simulink library "TM_MASTER"  (Simulink 8.6)
settings: Solver=ode45  StartTime=0.0  StopTime=10.0  RelTol=1e-3
libraries: cdsFilt x75, VIS_LIB x63, cdsEpicsOut x60, cdsTP x48, cdsMuxMatrix x17, cdsFiltCtrl x15, lockin x10, QPD x10, cdsRms x6, FOUROSEM_COILOUTF_MASTER x5, cdsFunctionCall x5, CRYP_TM_MASTER x3
(part 8 of 9)

== system TM_MASTER/TM_TYPEBP/ADD ==
  ISC_L_In : Inport
  ISC_P_In : Inport  Port=2
  ISC_Y_In : Inport  Port=3
  TEST_L_In : Inport  Port=4
  TEST_P_In : Inport  Port=5
  TEST_Y_In : Inport  Port=6
  DAMP_L_In : Inport  Port=7
  DAMP_P_In : Inport  Port=8
  DAMP_Y_In : Inport  Port=9
  Ground{1..6} (6 alike) : Ground
  L : cdsFiltCtrl/IIR FM with control  Tag=cdsFiltCtrl  Description=|
      | cdsFiltCntrl is the standard IIR filter module (exactly the same as cdsFilt) but with added control data output 'Ctrl'. Filter module digital signal output appears on the first output, which is called 'Val'. 'Ctrl' output has a bit pattern encoding the state of filter's on/off switches (FM1 through FM10). The bit values are:
      |                                                                                                                                                                                                                                                                                                                                       
      | module 	hex	dec                                                                                                                                                                                                                                                                                                                       
      | -----------------------                                                                                                                                                                                                                                                                                                               
      | FM1	0x20                    32                                                                                                                                                                                                                                                                                                        
      | FM2	0x80                     128                                                                                                                                                                                                                                                                                                      
      | FM3	0x200                   512                                                                                                                                                                                                                                                                                                       
      | FM4	0x800                   2048                                                                                                                                                                                                                                                                                                      
      | FM5	0x2000                 8192                                                                                                                                                                                                                                                                                                       
      | FM6	0x8000                 32768                                                                                                                                                                                                                                                                                                      
      | FM7	0x20000                131072                                                                                                                                                                                                                                                                                                     
      | FM8	0x80000                 524288                                                                                                                                                                                                                                                                                                    
      | FM9	0x200000               2097152                                                                                                                                                                                                                                                                                                    
      | FM10	0x800000               8388608                                                                                                                                                                                                                                                                                                   
      |                                                                                                                                                                                                                                                                                                                                       
      | This bit data can be used to drive some other switches or it can be output using a binary I/O module.
      settings: AttributesFormatString=%<Tag>
  P : cdsFiltCtrl/IIR FM with control  Tag=cdsFiltCtrl  Description=|
      | cdsFiltCntrl is the standard IIR filter module (exactly the same as cdsFilt) but with added control data output 'Ctrl'. Filter module digital signal output appears on the first output, which is called 'Val'. 'Ctrl' output has a bit pattern encoding the state of filter's on/off switches (FM1 through FM10). The bit values are:
      |                                                                                                                                                                                                                                                                                                                                       
      | module 	hex	dec                                                                                                                                                                                                                                                                                                                       
      | -----------------------                                                                                                                                                                                                                                                                                                               
      | FM1	0x20                    32                                                                                                                                                                                                                                                                                                        
      | FM2	0x80                     128                                                                                                                                                                                                                                                                                                      
      | FM3	0x200                   512                                                                                                                                                                                                                                                                                                       
      | FM4	0x800                   2048                                                                                                                                                                                                                                                                                                      
      | FM5	0x2000                 8192                                                                                                                                                                                                                                                                                                       
      | FM6	0x8000                 32768                                                                                                                                                                                                                                                                                                      
      | FM7	0x20000                131072                                                                                                                                                                                                                                                                                                     
      | FM8	0x80000                 524288                                                                                                                                                                                                                                                                                                    
      | FM9	0x200000               2097152                                                                                                                                                                                                                                                                                                    
      | FM10	0x800000               8388608                                                                                                                                                                                                                                                                                                   
      |                                                                                                                                                                                                                                                                                                                                       
      | This bit data can be used to drive some other switches or it can be output using a binary I/O module.
      settings: AttributesFormatString=%<Tag>
  Sum : Sum  Inputs=+++
  Sum3 : Sum  Inputs=+++
  Sum4 : Sum  Inputs=+++
  Terminator1 : Terminator
  Terminator2 : Terminator
  Terminator3 : Terminator
  Y : cdsFiltCtrl/IIR FM with control  Tag=cdsFiltCtrl  Description=|
      | cdsFiltCntrl is the standard IIR filter module (exactly the same as cdsFilt) but with added control data output 'Ctrl'. Filter module digital signal output appears on the first output, which is called 'Val'. 'Ctrl' output has a bit pattern encoding the state of filter's on/off switches (FM1 through FM10). The bit values are:
      |                                                                                                                                                                                                                                                                                                                                       
      | module 	hex	dec                                                                                                                                                                                                                                                                                                                       
      | -----------------------                                                                                                                                                                                                                                                                                                               
      | FM1	0x20                    32                                                                                                                                                                                                                                                                                                        
      | FM2	0x80                     128                                                                                                                                                                                                                                                                                                      
      | FM3	0x200                   512                                                                                                                                                                                                                                                                                                       
      | FM4	0x800                   2048                                                                                                                                                                                                                                                                                                      
      | FM5	0x2000                 8192                                                                                                                                                                                                                                                                                                       
      | FM6	0x8000                 32768                                                                                                                                                                                                                                                                                                      
      | FM7	0x20000                131072                                                                                                                                                                                                                                                                                                     
      | FM8	0x80000                 524288                                                                                                                                                                                                                                                                                                    
      | FM9	0x200000               2097152                                                                                                                                                                                                                                                                                                    
      | FM10	0x800000               8388608                                                                                                                                                                                                                                                                                                   
      |                                                                                                                                                                                                                                                                                                                                       
      | This bit data can be used to drive some other switches or it can be output using a binary I/O module.
      settings: AttributesFormatString=%<Tag>
  LONG_Out : Outport
  PITCH_Out : Outport  Port=2
  YAW_Out : Outport  Port=3
  wires:
  Y/2 -> Terminator3/1
  P/2 -> Terminator2/1
  L/2 -> Terminator1/1
  Y/1 -> YAW_Out/1
  Ground5/1 -> Y/2
  Ground4/1 -> Y/3
  Sum3/1 -> Y/1
  P/1 -> PITCH_Out/1
  Ground3/1 -> P/2
  Ground2/1 -> P/3
  Sum4/1 -> P/1
  L/1 -> LONG_Out/1
  Ground6/1 -> L/2
  Ground1/1 -> L/3
  Sum/1 -> L/1
  ISC_P_In/1 -> Sum4/1
  TEST_P_In/1 -> Sum4/2
  TEST_Y_In/1 -> Sum3/2
  ISC_Y_In/1 -> Sum3/1
  TEST_L_In/1 -> Sum/2
  ISC_L_In/1 -> Sum/1
  DAMP_L_In/1 -> Sum/3
  DAMP_P_In/1 -> Sum4/3
  DAMP_Y_In/1 -> Sum3/3

== system TM_MASTER/TM_TYPEBP/ADDASC ==
  ISC_P_In : Inport
  ISC_Y_In : Inport  Port=2
  DITHER_P_In : Inport  Port=3
  DITHER_Y_In : Inport  Port=4
  Sum3 : Sum
  Sum4 : Sum
  PITCH_Out : Outport
  YAW_Out : Outport  Port=2
  wires:
  Sum3/1 -> YAW_Out/1
  ISC_P_In/1 -> Sum4/1
  ISC_Y_In/1 -> Sum3/1
  Sum4/1 -> PITCH_Out/1
  DITHER_P_In/1 -> Sum4/2
  DITHER_Y_In/1 -> Sum3/2

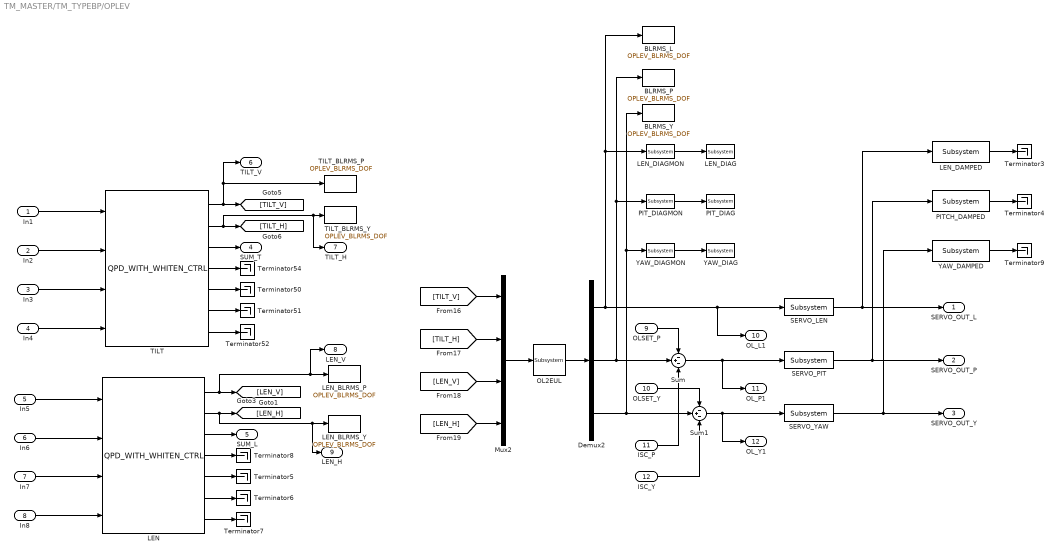
== system TM_MASTER/TM_TYPEBP/OPLEV ==
  In1 : Inport
  In2 : Inport  Port=2
  In3 : Inport  Port=3
  In4 : Inport  Port=4
  In5 : Inport  Port=5
  In6 : Inport  Port=6
  In7 : Inport  Port=7
  In8 : Inport  Port=8
  OLSET_P : Inport  Port=9
  OLSET_Y : Inport  Port=10
  ISC_P : Inport  Port=11
  ISC_Y : Inport  Port=12
  BLRMS_L : VIS_LIB/OPLEV_BLRMS_DOF
  BLRMS_P : VIS_LIB/OPLEV_BLRMS_DOF
  BLRMS_Y : VIS_LIB/OPLEV_BLRMS_DOF
  Demux2 : Demux  Outputs=3
  LEN : QPD/QPD_WITH_WHITEN_CTRL
  LEN_BLRMS_P : VIS_LIB/OPLEV_BLRMS_DOF
  LEN_BLRMS_Y : VIS_LIB/OPLEV_BLRMS_DOF
  LEN_DAMPED : cdsEpicsOut/Subsystem  Tag=cdsEpicsOutput  Description=|
      | Purpose:                                          
      | Output a FE signal to an EPICS channel.           
      |                                                   
      | Operation:                                        
      | Takes input value and passes it to EPICS record.  
      |                                                   
      | Usage:                                            
      | Name the part with the desired EPICS rrecord name.
      settings: AttributesFormatString=%<Tag>
  LEN_DIAG : cdsTP/Subsystem  Tag=Test Point
      settings: AttributesFormatString=%<Tag>
  LEN_DIAGMON : cdsEpicsOut/Subsystem  Tag=cdsEpicsOutput  Description=|
      | Purpose:                                          
      | Output a FE signal to an EPICS channel.           
      |                                                   
      | Operation:                                        
      | Takes input value and passes it to EPICS record.  
      |                                                   
      | Usage:                                            
      | Name the part with the desired EPICS rrecord name.
      settings: AttributesFormatString=%<Tag>
  Mux2 : Mux
  OL2EUL : cdsMuxMatrix/Subsystem  Tag=cdsMuxMatrix  Description=Any size matrix. Inputs and outputs must be connected using Mux and Demux parts.
      settings: AttributesFormatString=%<Tag>
  PITCH_DAMPED : cdsEpicsOut/Subsystem  Tag=cdsEpicsOutput  Description=|
      | Purpose:                                          
      | Output a FE signal to an EPICS channel.           
      |                                                   
      | Operation:                                        
      | Takes input value and passes it to EPICS record.  
      |                                                   
      | Usage:                                            
      | Name the part with the desired EPICS rrecord name.
      settings: AttributesFormatString=%<Tag>
  PIT_DIAG : cdsTP/Subsystem  Tag=Test Point
      settings: AttributesFormatString=%<Tag>
  PIT_DIAGMON : cdsEpicsOut/Subsystem  Tag=cdsEpicsOutput  Description=|
      | Purpose:                                          
      | Output a FE signal to an EPICS channel.           
      |                                                   
      | Operation:                                        
      | Takes input value and passes it to EPICS record.  
      |                                                   
      | Usage:                                            
      | Name the part with the desired EPICS rrecord name.
      settings: AttributesFormatString=%<Tag>
  SERVO_LEN : cdsFilt/Subsystem  Tag=cdsFilt  Description=|
      | Purpose:                                                                                                                                                                                                                                  
      | Standard CDS IIR filter module.                                                                                                                                                                                                           
      |                                                                                                                                                                                                                                           
      | Operation:                                                                                                                                                                                                                                
      | Consists of 10 second order section IIR filters, plus a ramped gain stage. In FE code, also provides pre-defined test points and excitation channel inputs. The filter coefficients are defined in the LIGO system using the 'foton' tool.
      |                                                                                                                                                                                                                                           
      | Usage:                                                                                                                                                                                                                                    
      | Name the part with the desired filter module name.
      settings: AttributesFormatString=%<Tag>
  SERVO_PIT : cdsFilt/Subsystem  Tag=cdsFilt  Description=|
      | Purpose:                                                                                                                                                                                                                                  
      | Standard CDS IIR filter module.                                                                                                                                                                                                           
      |                                                                                                                                                                                                                                           
      | Operation:                                                                                                                                                                                                                                
      | Consists of 10 second order section IIR filters, plus a ramped gain stage. In FE code, also provides pre-defined test points and excitation channel inputs. The filter coefficients are defined in the LIGO system using the 'foton' tool.
      |                                                                                                                                                                                                                                           
      | Usage:                                                                                                                                                                                                                                    
      | Name the part with the desired filter module name.
      settings: AttributesFormatString=%<Tag>
  SERVO_YAW : cdsFilt/Subsystem  Tag=cdsFilt  Description=|
      | Purpose:                                                                                                                                                                                                                                  
      | Standard CDS IIR filter module.                                                                                                                                                                                                           
      |                                                                                                                                                                                                                                           
      | Operation:                                                                                                                                                                                                                                
      | Consists of 10 second order section IIR filters, plus a ramped gain stage. In FE code, also provides pre-defined test points and excitation channel inputs. The filter coefficients are defined in the LIGO system using the 'foton' tool.
      |                                                                                                                                                                                                                                           
      | Usage:                                                                                                                                                                                                                                    
      | Name the part with the desired filter module name.
      settings: AttributesFormatString=%<Tag>
  Sum : Sum  Inputs=-+-
  Sum1 : Sum  Inputs=-+-
  TILT : QPD/QPD_WITH_WHITEN_CTRL
  TILT_BLRMS_P : VIS_LIB/OPLEV_BLRMS_DOF
  TILT_BLRMS_Y : VIS_LIB/OPLEV_BLRMS_DOF
  Terminator{3..9,50..52,54} (11 alike) : Terminator
  YAW_DAMPED : cdsEpicsOut/Subsystem  Tag=cdsEpicsOutput  Description=|
      | Purpose:                                          
      | Output a FE signal to an EPICS channel.           
      |                                                   
      | Operation:                                        
      | Takes input value and passes it to EPICS record.  
      |                                                   
      | Usage:                                            
      | Name the part with the desired EPICS rrecord name.
      settings: AttributesFormatString=%<Tag>
  YAW_DIAG : cdsTP/Subsystem  Tag=Test Point
      settings: AttributesFormatString=%<Tag>
  YAW_DIAGMON : cdsEpicsOut/Subsystem  Tag=cdsEpicsOutput  Description=|
      | Purpose:                                          
      | Output a FE signal to an EPICS channel.           
      |                                                   
      | Operation:                                        
      | Takes input value and passes it to EPICS record.  
      |                                                   
      | Usage:                                            
      | Name the part with the desired EPICS rrecord name.
      settings: AttributesFormatString=%<Tag>
  SERVO_OUT_L : Outport
  SERVO_OUT_P : Outport  Port=2
  SERVO_OUT_Y : Outport  Port=3
  SUM_T : Outport  Port=4
  SUM_L : Outport  Port=5
  TILT_V : Outport  Port=6
  TILT_H : Outport  Port=7
  LEN_V : Outport  Port=8
  LEN_H : Outport  Port=9
  OL_L1 : Outport  Port=10
  OL_P1 : Outport  Port=11
  OL_Y1 : Outport  Port=12
  wires:
  [LEN_H] -> Mux2/4
  Mux2/1 -> OL2EUL/1
  TILT/5 -> Terminator50/1
  TILT/7 -> Terminator52/1
  TILT/6 -> Terminator51/1
  TILT/4 -> Terminator54/1
  TILT/3 -> SUM_T/1
  TILT/1 -> TILT_V/1, TILT_BLRMS_P/1, [TILT_V]
  TILT/2 -> TILT_H/1, TILT_BLRMS_Y/1, [TILT_H]
  In4/1 -> TILT/4
  In3/1 -> TILT/3
  In2/1 -> TILT/2
  In1/1 -> TILT/1
  OL2EUL/1 -> Demux2/1
  In7/1 -> LEN/3
  In6/1 -> LEN/2
  In5/1 -> LEN/1
  [LEN_V] -> Mux2/3
  LEN/3 -> SUM_L/1
  LEN/1 -> LEN_V/1, LEN_BLRMS_P/1, [LEN_V]
  In8/1 -> LEN/4
  [TILT_V] -> Mux2/1
  LEN/7 -> Terminator7/1
  LEN/6 -> Terminator6/1
  LEN/5 -> Terminator5/1
  LEN/4 -> Terminator8/1
  [TILT_H] -> Mux2/2
  Demux2/2 -> Sum/2, PIT_DIAGMON/1, BLRMS_P/1
  Demux2/3 -> Sum1/2, BLRMS_Y/1, YAW_DIAGMON/1
  SERVO_LEN/1 -> LEN_DAMPED/1, SERVO_OUT_L/1
  SERVO_PIT/1 -> PITCH_DAMPED/1, SERVO_OUT_P/1
  SERVO_YAW/1 -> YAW_DAMPED/1, SERVO_OUT_Y/1
  LEN_DAMPED/1 -> Terminator3/1
  PITCH_DAMPED/1 -> Terminator4/1
  YAW_DAMPED/1 -> Terminator9/1
  LEN_DIAGMON/1 -> LEN_DIAG/1
  PIT_DIAGMON/1 -> PIT_DIAG/1
  YAW_DIAGMON/1 -> YAW_DIAG/1
  LEN/2 -> [LEN_H], LEN_H/1, LEN_BLRMS_Y/1
  OLSET_Y/1 -> Sum1/1
  OLSET_P/1 -> Sum/1
  ISC_P/1 -> Sum/3
  ISC_Y/1 -> Sum1/3
  Demux2/1 -> BLRMS_L/1, LEN_DIAGMON/1, OL_L1/1, SERVO_LEN/1
  Sum/1 -> OL_P1/1, SERVO_PIT/1
  Sum1/1 -> OL_Y1/1, SERVO_YAW/1

== system TM_MASTER/TM_TYPEBP/TEST ==
  Ground : Ground
  Ground1 : Ground
  Ground2 : Ground
  L : cdsFilt/Subsystem  Tag=cdsFilt  Description=|
      | Purpose:                                                                                                                                                                                                                                  
      | Standard CDS IIR filter module.                                                                                                                                                                                                           
      |                                                                                                                                                                                                                                           
      | Operation:                                                                                                                                                                                                                                
      | Consists of 10 second order section IIR filters, plus a ramped gain stage. In FE code, also provides pre-defined test points and excitation channel inputs. The filter coefficients are defined in the LIGO system using the 'foton' tool.
      |                                                                                                                                                                                                                                           
      | Usage:                                                                                                                                                                                                                                    
      | Name the part with the desired filter module name.
      settings: AttributesFormatString=%<Tag>
  P : cdsFilt/Subsystem  Tag=cdsFilt  Description=|
      | Purpose:                                                                                                                                                                                                                                  
      | Standard CDS IIR filter module.                                                                                                                                                                                                           
      |                                                                                                                                                                                                                                           
      | Operation:                                                                                                                                                                                                                                
      | Consists of 10 second order section IIR filters, plus a ramped gain stage. In FE code, also provides pre-defined test points and excitation channel inputs. The filter coefficients are defined in the LIGO system using the 'foton' tool.
      |                                                                                                                                                                                                                                           
      | Usage:                                                                                                                                                                                                                                    
      | Name the part with the desired filter module name.
      settings: AttributesFormatString=%<Tag>
  Y : cdsFilt/Subsystem  Tag=cdsFilt  Description=|
      | Purpose:                                                                                                                                                                                                                                  
      | Standard CDS IIR filter module.                                                                                                                                                                                                           
      |                                                                                                                                                                                                                                           
      | Operation:                                                                                                                                                                                                                                
      | Consists of 10 second order section IIR filters, plus a ramped gain stage. In FE code, also provides pre-defined test points and excitation channel inputs. The filter coefficients are defined in the LIGO system using the 'foton' tool.
      |                                                                                                                                                                                                                                           
      | Usage:                                                                                                                                                                                                                                    
      | Name the part with the desired filter module name.
      settings: AttributesFormatString=%<Tag>
  LONG_Out : Outport
  PITCH_Out : Outport  Port=2
  YAW_Out : Outport  Port=3
  wires:
  P/1 -> PITCH_Out/1
  Y/1 -> YAW_Out/1
  L/1 -> LONG_Out/1
  Ground1/1 -> P/1
  Ground/1 -> L/1
  Ground2/1 -> Y/1

== system TM_MASTER/PHASE1_TM/WD/OLAC ==
  T_In : Inport
  L_In : Inport  Port=2
  Abs1 : Abs
  Abs2 : Abs
  BANDLIM : Subsystem
  LRMS : cdsRms/Subsystem  Tag=cdsRms  Description=|
      | Purpose:
      | Calculate an RMS based on the input signal.
      settings: AttributesFormatString=%<Tag>
  L_RMS : cdsTP/Subsystem  Tag=Test Point
      settings: AttributesFormatString=%<Tag>
  L_RMSMON : cdsEpicsOut/Subsystem  Tag=cdsEpicsOutput  Description=|
      | Purpose:                                          
      | Output a FE signal to an EPICS channel.           
      |                                                   
      | Operation:                                        
      | Takes input value and passes it to EPICS record.  
      |                                                   
      | Usage:                                            
      | Name the part with the desired EPICS rrecord name.
      settings: AttributesFormatString=%<Tag>
  Operator1 : RelationalOperator  Operator=>  OutDataTypeStr=boolean
  Operator2 : RelationalOperator  Operator=>  OutDataTypeStr=boolean
  RMS_MAX : cdsEpicsIn/Subsystem  Tag=cdsEpicsIn  Description=|
      | Purpose:                                                                              
      | Create an EPICS input channel connection to the FE realtime controls.                 
      |                                                                                       
      | Operation:                                                                            
      | Outputs value from an EPICS ai record. Value is floating point with a precision of 3..
      |                                                                                       
      | Usage:                                                                                
      | Name the part with the desired EPICS channel name.
      settings: AttributesFormatString=%<Tag>
  Sum1 : Sum
  TRMS : cdsRms/Subsystem  Tag=cdsRms  Description=|
      | Purpose:
      | Calculate an RMS based on the input signal.
      settings: AttributesFormatString=%<Tag>
  T_RMS : cdsTP/Subsystem  Tag=Test Point
      settings: AttributesFormatString=%<Tag>
  T_RMSMON : cdsEpicsOut/Subsystem  Tag=cdsEpicsOutput  Description=|
      | Purpose:                                          
      | Output a FE signal to an EPICS channel.           
      |                                                   
      | Operation:                                        
      | Takes input value and passes it to EPICS record.  
      |                                                   
      | Usage:                                            
      | Name the part with the desired EPICS rrecord name.
      settings: AttributesFormatString=%<Tag>
  FLAG : Outport
  wires:
  Abs1/1 -> Operator1/2
  BANDLIM/2(L_Out) -> LRMS/1
  BANDLIM/1(T_Out) -> TRMS/1
  L_In/1 -> BANDLIM/2(L_In)
  T_In/1 -> BANDLIM/1(T_In)
  L_RMSMON/1 -> Abs2/1
  T_RMSMON/1 -> Abs1/1
  Operator1/1 -> Sum1/1
  Operator2/1 -> Sum1/2
  Abs2/1 -> Operator2/2
  RMS_MAX/1 -> Operator2/1, Operator1/1
  LRMS/1 -> L_RMS/1, L_RMSMON/1
  TRMS/1 -> T_RMS/1, T_RMSMON/1
  Sum1/1 -> FLAG/1

== system TM_MASTER/PHASE1_TM_NEW/WD/OLAC ==
  T_In : Inport
  L_In : Inport  Port=2
  Abs1 : Abs
  Abs2 : Abs
  BANDLIM : Subsystem
  LRMS : cdsRms/Subsystem  Tag=cdsRms  Description=|
      | Purpose:
      | Calculate an RMS based on the input signal.
      settings: AttributesFormatString=%<Tag>
  L_RMS : cdsTP/Subsystem  Tag=Test Point
      settings: AttributesFormatString=%<Tag>
  L_RMSMON : cdsEpicsOut/Subsystem  Tag=cdsEpicsOutput  Description=|
      | Purpose:                                          
      | Output a FE signal to an EPICS channel.           
      |                                                   
      | Operation:                                        
      | Takes input value and passes it to EPICS record.  
      |                                                   
      | Usage:                                            
      | Name the part with the desired EPICS rrecord name.
      settings: AttributesFormatString=%<Tag>
  Operator1 : RelationalOperator  Operator=>  OutDataTypeStr=boolean
  Operator2 : RelationalOperator  Operator=>  OutDataTypeStr=boolean
  RMS_MAX : cdsEpicsIn/Subsystem  Tag=cdsEpicsIn  Description=|
      | Purpose:                                                                              
      | Create an EPICS input channel connection to the FE realtime controls.                 
      |                                                                                       
      | Operation:                                                                            
      | Outputs value from an EPICS ai record. Value is floating point with a precision of 3..
      |                                                                                       
      | Usage:                                                                                
      | Name the part with the desired EPICS channel name.
      settings: AttributesFormatString=%<Tag>
  Sum1 : Sum
  TRMS : cdsRms/Subsystem  Tag=cdsRms  Description=|
      | Purpose:
      | Calculate an RMS based on the input signal.
      settings: AttributesFormatString=%<Tag>
  T_RMS : cdsTP/Subsystem  Tag=Test Point
      settings: AttributesFormatString=%<Tag>
  T_RMSMON : cdsEpicsOut/Subsystem  Tag=cdsEpicsOutput  Description=|
      | Purpose:                                          
      | Output a FE signal to an EPICS channel.           
      |                                                   
      | Operation:                                        
      | Takes input value and passes it to EPICS record.  
      |                                                   
      | Usage:                                            
      | Name the part with the desired EPICS rrecord name.
      settings: AttributesFormatString=%<Tag>
  FLAG : Outport
  wires:
  Abs1/1 -> Operator1/2
  BANDLIM/2(L_Out) -> LRMS/1
  BANDLIM/1(T_Out) -> TRMS/1
  L_In/1 -> BANDLIM/2(L_In)
  T_In/1 -> BANDLIM/1(T_In)
  L_RMSMON/1 -> Abs2/1
  T_RMSMON/1 -> Abs1/1
  Operator1/1 -> Sum1/1
  Operator2/1 -> Sum1/2
  Abs2/1 -> Operator2/2
  RMS_MAX/1 -> Operator2/1, Operator1/1
  LRMS/1 -> L_RMS/1, L_RMSMON/1
  TRMS/1 -> T_RMS/1, T_RMSMON/1
  Sum1/1 -> FLAG/1

== system TM_MASTER/TM/WD/OLAC ==
  T_In : Inport
  L_In : Inport  Port=2
  Abs1 : Abs
  Abs2 : Abs
  BANDLIM : Subsystem
  LRMS : cdsRms/Subsystem  Tag=cdsRms  Description=|
      | Purpose:
      | Calculate an RMS based on the input signal.
      settings: AttributesFormatString=%<Tag>
  L_RMS : cdsTP/Subsystem  Tag=Test Point
      settings: AttributesFormatString=%<Tag>
  L_RMSMON : cdsEpicsOut/Subsystem  Tag=cdsEpicsOutput  Description=|
      | Purpose:                                          
      | Output a FE signal to an EPICS channel.           
      |                                                   
      | Operation:                                        
      | Takes input value and passes it to EPICS record.  
      |                                                   
      | Usage:                                            
      | Name the part with the desired EPICS rrecord name.
      settings: AttributesFormatString=%<Tag>
  Operator1 : RelationalOperator  Operator=>  OutDataTypeStr=boolean
  Operator2 : RelationalOperator  Operator=>  OutDataTypeStr=boolean
  RMS_MAX : cdsEpicsIn/Subsystem  Tag=cdsEpicsIn  Description=|
      | Purpose:                                                                              
      | Create an EPICS input channel connection to the FE realtime controls.                 
      |                                                                                       
      | Operation:                                                                            
      | Outputs value from an EPICS ai record. Value is floating point with a precision of 3..
      |                                                                                       
      | Usage:                                                                                
      | Name the part with the desired EPICS channel name.
      settings: AttributesFormatString=%<Tag>
  Sum1 : Sum
  TRMS : cdsRms/Subsystem  Tag=cdsRms  Description=|
      | Purpose:
      | Calculate an RMS based on the input signal.
      settings: AttributesFormatString=%<Tag>
  T_RMS : cdsTP/Subsystem  Tag=Test Point
      settings: AttributesFormatString=%<Tag>
  T_RMSMON : cdsEpicsOut/Subsystem  Tag=cdsEpicsOutput  Description=|
      | Purpose:                                          
      | Output a FE signal to an EPICS channel.           
      |                                                   
      | Operation:                                        
      | Takes input value and passes it to EPICS record.  
      |                                                   
      | Usage:                                            
      | Name the part with the desired EPICS rrecord name.
      settings: AttributesFormatString=%<Tag>
  FLAG : Outport
  wires:
  Abs1/1 -> Operator1/2
  BANDLIM/2(L_Out) -> LRMS/1
  BANDLIM/1(T_Out) -> TRMS/1
  L_In/1 -> BANDLIM/2(L_In)
  T_In/1 -> BANDLIM/1(T_In)
  L_RMSMON/1 -> Abs2/1
  T_RMSMON/1 -> Abs1/1
  Operator1/1 -> Sum1/1
  Operator2/1 -> Sum1/2
  Abs2/1 -> Operator2/2
  RMS_MAX/1 -> Operator2/1, Operator1/1
  LRMS/1 -> L_RMS/1, L_RMSMON/1
  TRMS/1 -> T_RMS/1, T_RMSMON/1
  Sum1/1 -> FLAG/1

== system TM_MASTER/PHASE1_TM/WD/OLAC/BANDLIM ==
  T_In : Inport
  L_In : Inport  Port=2
  L : cdsFilt/Subsystem  Tag=cdsFilt  Description=|
      | Purpose:                                                                                                                                                                                                                                  
      | Standard CDS IIR filter module.                                                                                                                                                                                                           
      |                                                                                                                                                                                                                                           
      | Operation:                                                                                                                                                                                                                                
      | Consists of 10 second order section IIR filters, plus a ramped gain stage. In FE code, also provides pre-defined test points and excitation channel inputs. The filter coefficients are defined in the LIGO system using the 'foton' tool.
      |                                                                                                                                                                                                                                           
      | Usage:                                                                                                                                                                                                                                    
      | Name the part with the desired filter module name.
      settings: AttributesFormatString=%<Tag>
  T : cdsFilt/Subsystem  Tag=cdsFilt  Description=|
      | Purpose:                                                                                                                                                                                                                                  
      | Standard CDS IIR filter module.                                                                                                                                                                                                           
      |                                                                                                                                                                                                                                           
      | Operation:                                                                                                                                                                                                                                
      | Consists of 10 second order section IIR filters, plus a ramped gain stage. In FE code, also provides pre-defined test points and excitation channel inputs. The filter coefficients are defined in the LIGO system using the 'foton' tool.
      |                                                                                                                                                                                                                                           
      | Usage:                                                                                                                                                                                                                                    
      | Name the part with the desired filter module name.
      settings: AttributesFormatString=%<Tag>
  T_Out : Outport
  L_Out : Outport  Port=2
  wires:
  L_In/1 -> L/1
  T_In/1 -> T/1
  L/1 -> L_Out/1
  T/1 -> T_Out/1
